simulink model "RTLAB_Sim_HVandLV_2015B"  (R2015b)
settings: Solver=ode45  StartTime=0.0  StopTime=20  RelTol=1e-3
values from neighbouring files (symbols this model uses):
  Ts = 20e-6    (= 2e-05)    [DataPostProcess.m]    (also in PlotData.m = 5e-05; data_analysis_01_MAT_load.m; data_analysis_01_Plot_result.m = 5e-05; data_analysis_02_Postprocess_Batch.m)
  Vrms_ph_hv = 37e3    (= 37000)    [DataPostProcess.m]    (also in data_analysis_01_MAT_load.m; data_analysis_05_Postprocess_Batch.m)
  Vrms_ph_lv = 690    [DataPostProcess.m]    (also in data_analysis_01_MAT_load.m; data_analysis_05_Postprocess_Batch.m)
libraries: powerlib_extras x5, powerlib_meascontrol x4, powerlib x1
settings Model: SimulationMode=accelerator  Creator=keliang  LastModifiedBy=anony
settings DataIOCC: SaveFormat=Array
settings OptimizationCC: EfficientMapNaN2IntZero=off
settings DebuggingCC: AllowSymbolicDim=on
settings HardwareCC: ProdWordSize=32  ProdHWDeviceType=Specified  TargetBitPerPointer=64  TargetLongLongMode=on  TargetIntDivRoundTo=Zero  TargetEndianess=LittleEndian  TargetWordSize=64  TargetHWDeviceType=MATLAB Host  ProdEqTarget=off
settings CodeAppCC: MaxIdLength=128
settings GRTTargetCC: CombineOutputUpdateFcns=off  GRTInterface=on
settings ConfigComp: CovModelRefEnable=Off
settings ConfigurationSet: Description=Simscape Multibody

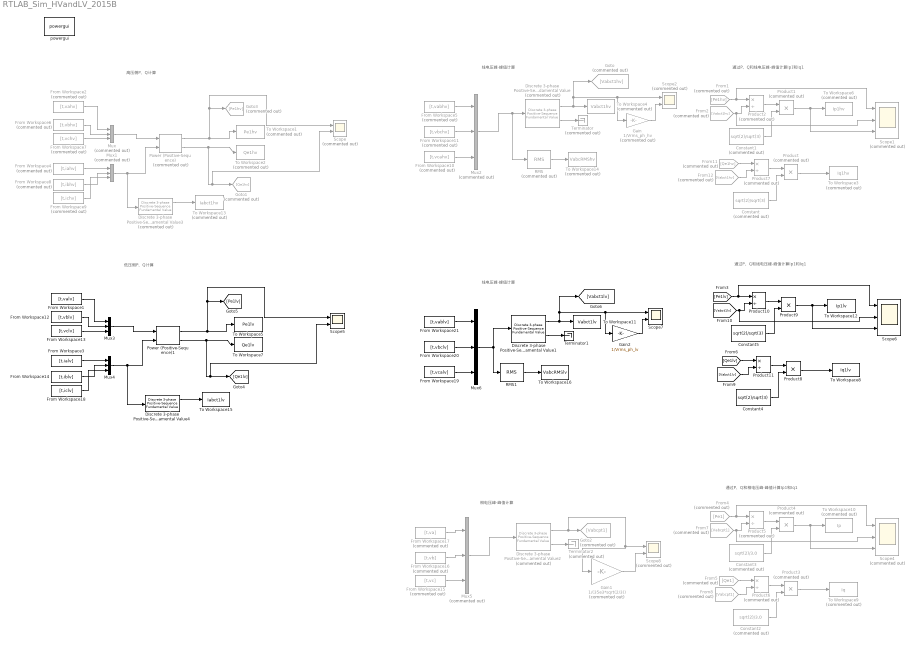
== system RTLAB_Sim_HVandLV_2015B ==
  note: 相电压峰-峰值计算
  note: 线电压峰-峰值计算
  note: 高压侧P、Q计算
  note: 通过P、Q和线电压峰-峰值计算Ip1和Iq1
  note: 通过P、Q和相电压峰-峰值计算Ip1和Iq1
  note: 低压侧P、Q计算
  note: 线电压峰-峰值计算
  note: 通过P、Q和线电压峰-峰值计算Ip1和Iq1
  Constant : Constant  Commented=on  Value=sqrt(2)/sqrt(3)
  Constant1 : Constant  Commented=on  Value=sqrt(2)/sqrt(3)
  Constant2 : Constant  Commented=on  Value=sqrt(2)/3.0
  Constant3 : Constant  Commented=on  Value=sqrt(2)/3.0
  Constant4 : Constant  Value=sqrt(2)/sqrt(3)
  Constant5 : Constant  Value=sqrt(2)/sqrt(3)
  Discrete 3-phase Positive-Sequence Fundamental Value : powerlib_extras/Discrete Measurements/Discrete 3-phase Positive-Sequence Fundamental Value  Commented=on  Freq=50  Par_Init=[0 0]  Ts=Ts
  Discrete 3-phase Positive-Sequence Fundamental Value1 : powerlib_extras/Discrete Measurements/Discrete 3-phase Positive-Sequence Fundamental Value  Freq=50  Par_Init=[0 0]  Ts=Ts
  Discrete 3-phase Positive-Sequence Fundamental Value2 : powerlib_extras/Discrete Measurements/Discrete 3-phase Positive-Sequence Fundamental Value  Commented=on  Freq=50  Par_Init=[0 0]  Ts=Ts
  Discrete 3-phase Positive-Sequence Fundamental Value3 : powerlib_extras/Discrete Measurements/Discrete 3-phase Positive-Sequence Fundamental Value  Commented=on  Freq=50  Par_Init=[0 0]  Ts=Ts
  Discrete 3-phase Positive-Sequence Fundamental Value4 : powerlib_extras/Discrete Measurements/Discrete 3-phase Positive-Sequence Fundamental Value  Freq=100  Par_Init=[0 0]  Ts=Ts
  From Workspace1 : FromWorkspace  VariableName=[t,valv]
  From Workspace10 : FromWorkspace  Commented=on  VariableName=[t,vcahv]
  From Workspace11 : FromWorkspace  Commented=on  VariableName=[t,vbchv]
  From Workspace12 : FromWorkspace  VariableName=[t,vblv]
  From Workspace13 : FromWorkspace  VariableName=[t,vclv]
  From Workspace14 : FromWorkspace  VariableName=[t,iblv]
  From Workspace15 : FromWorkspace  Commented=on  VariableName=[t,vc]
  From Workspace16 : FromWorkspace  Commented=on  VariableName=[t,vb]
  From Workspace17 : FromWorkspace  Commented=on  VariableName=[t,va]
  From Workspace18 : FromWorkspace  VariableName=[t,iclv]
  From Workspace19 : FromWorkspace  VariableName=[t,vcalv]
  From Workspace2 : FromWorkspace  Commented=on  VariableName=[t,vahv]
  From Workspace20 : FromWorkspace  VariableName=[t,vbclv]
  From Workspace21 : FromWorkspace  VariableName=[t,vablv]
  From Workspace3 : FromWorkspace  VariableName=[t,ialv]
  From Workspace4 : FromWorkspace  Commented=on  VariableName=[t,iahv]
  From Workspace5 : FromWorkspace  Commented=on  VariableName=[t,vabhv]
  From Workspace6 : FromWorkspace  Commented=on  VariableName=[t,vbhv]
  From Workspace7 : FromWorkspace  Commented=on  VariableName=[t,vchv]
  From Workspace8 : FromWorkspace  Commented=on  VariableName=[t,ibhv]
  From Workspace9 : FromWorkspace  Commented=on  VariableName=[t,ichv]
  From1 : From  Commented=on  GotoTag=Pe1hv
      settings: CloseFcn=tagdialog Close
  From11 : From  Commented=on  GotoTag=Qe1hv
      settings: CloseFcn=tagdialog Close
  From12 : From  Commented=on  GotoTag=Vabct1hv
      settings: CloseFcn=tagdialog Close
  From2 : From  Commented=on  GotoTag=Vabct1hv
      settings: CloseFcn=tagdialog Close
  From4 : From  Commented=on  GotoTag=Pe1
      settings: CloseFcn=tagdialog Close
  From5 : From  Commented=on  GotoTag=Qe1
      settings: CloseFcn=tagdialog Close
  From7 : From  Commented=on  GotoTag=Vabcpt1
      settings: CloseFcn=tagdialog Close
  From8 : From  Commented=on  GotoTag=Vabcpt1
      settings: CloseFcn=tagdialog Close
  Gain : Gain  Commented=on  Gain=1/Vrms_ph_hv
  Gain1 : Gain  Commented=on  Gain=1/(35e3*sqrt(2/3))
  Gain2 : Gain  Gain=1/Vrms_ph_lv
  Goto : Goto  Commented=on  GotoTag=Vabct1hv
  Goto1 : Goto  Commented=on  GotoTag=Qe1hv
  Goto2 : Goto  Commented=on  GotoTag=Vabcpt1
  Goto3 : Goto  Commented=on  GotoTag=Pe1hv
  Mux{,1..2,5} (4 alike) : Mux  Commented=on  Inputs=3
  Mux3 : Mux  Inputs=3
  Mux4 : Mux  Inputs=3
  Mux6 : Mux  Inputs=3
  Power (Positive-Sequence) : powerlib_meascontrol/Measurements/Power (Positive-Sequence)  Commented=on  Freq=50  Vinit=[0, 0]  Iinit=[0, 0]  Ts=Ts
  Power (Positive-Sequence)1 : powerlib_meascontrol/Measurements/Power (Positive-Sequence)  Freq=50  Vinit=[0, 0]  Iinit=[0, 0]  Ts=Ts
  Product{,1,3..4} (4 alike) : Product  Commented=on
  Product10 : Product  Inputs=*/  RndMeth=Zero
  Product11 : Product  Inputs=*/  RndMeth=Zero
  Product{2,5..7} (4 alike) : Product  Commented=on  Inputs=*/  RndMeth=Zero
  Product8 : Product
  Product9 : Product
  RMS : powerlib_meascontrol/Measurements/RMS  Commented=on  TrueRMS=on  Freq=100  RMSInit=0  Ts=Ts
  RMS1 : powerlib_meascontrol/Measurements/RMS  TrueRMS=on  Freq=100  RMSInit=0  Ts=Ts
  Scope : Scope  Commented=on  NumInputPorts=2
  Scope1 : Scope  Commented=on  NumInputPorts=3
  Scope2 : Scope  Commented=on  NumInputPorts=2
  Scope4 : Scope  Commented=on  NumInputPorts=3
  Scope5 : Scope  NumInputPorts=2
  Scope6 : Scope  NumInputPorts=3
  Scope7 : Scope  NumInputPorts=2
  Scope8 : Scope  Commented=on  NumInputPorts=2
  Terminator : Terminator  Commented=on
  Terminator1 : Terminator
  Terminator2 : Terminator  Commented=on
  To Workspace1 : ToWorkspace  Commented=on  VariableName=Pe1hv  SaveFormat=Structure With Time  SampleTime=-1
  To Workspace10 : ToWorkspace  Commented=on  VariableName=Ip  SaveFormat=Structure With Time  SampleTime=-1
  To Workspace11 : ToWorkspace  VariableName=Vabct1lv  SaveFormat=Structure With Time  SampleTime=-1
  To Workspace12 : ToWorkspace  VariableName=Ip1lv  SaveFormat=Structure With Time  SampleTime=-1
  To Workspace13 : ToWorkspace  Commented=on  VariableName=Iabct1hv  SaveFormat=Structure With Time  SampleTime=-1
  To Workspace14 : ToWorkspace  Commented=on  VariableName=VabcRMShv  SaveFormat=Structure With Time  SampleTime=-1
  To Workspace15 : ToWorkspace  VariableName=Iabct1lv  SaveFormat=Structure With Time  SampleTime=-1
  To Workspace16 : ToWorkspace  VariableName=VabcRMSlv  SaveFormat=Structure With Time  SampleTime=-1
  To Workspace2 : ToWorkspace  Commented=on  VariableName=Qe1hv  SaveFormat=Structure With Time  SampleTime=-1
  To Workspace3 : ToWorkspace  Commented=on  VariableName=Iq1hv  SaveFormat=Structure With Time  SampleTime=-1
  To Workspace4 : ToWorkspace  Commented=on  VariableName=Vabct1hv  SaveFormat=Structure With Time  SampleTime=-1
  To Workspace5 : ToWorkspace  VariableName=Pe1lv  SaveFormat=Structure With Time  SampleTime=-1
  To Workspace6 : ToWorkspace  Commented=on  VariableName=Ip1hv  SaveFormat=Structure With Time  SampleTime=-1
  To Workspace7 : ToWorkspace  VariableName=Qe1lv  SaveFormat=Structure With Time  SampleTime=-1
  To Workspace8 : ToWorkspace  VariableName=Iq1lv  SaveFormat=Structure With Time  SampleTime=-1
  To Workspace9 : ToWorkspace  Commented=on  VariableName=Iq  SaveFormat=Structure With Time  SampleTime=-1
  powergui : powerlib/powergui  Priority=1  SimulationMode=Discrete  SampleTime=Ts  frequency=60  Iterations=50  frequencyindice=60  Pbase=100e6  ErrMax=1e-4  UnitsV=kV  UnitsW=MW  buscounter=0  FunctionMessages=off  echomessages=off  EnableUseOfTLC=off  CurrentSourceSwitches=off  DisableSnubberDevices=off  DisableRonSwitches=off  DisableVfSwitches=off  DisplayEquations=off  AutomaticDiscreteSolvers=off  SolverType=Tustin  Interpol=off  ExternalGateDelay=off  methode=off  Ts=10  x0status=blocks  SPID=off  SwTol=0  HookPort=off  NonlinearTolerance=1e-4  nMaxIteration=100  ContinueOnMaxIteration=off  RestoreLinks=warning  ResistiveCurrentMeasurement=off  Frange=[0:2:500]  Ylog=off  Xlog=on  ShowGrid=off  save=off  variable=ZData  structure=v1  ZoomFFT=off  StartTime=3  cycles=50  DisplayStyle=1  fundamental=50  FreqAxis=off  MaxFrequency=2000  frequencyindicesteady=1  RmsSteady=1  display=off
  wires:
  Power (Positive-Sequence)/1 -> Scope/1, Goto3/1, To Workspace1/1
  Power (Positive-Sequence)/2 -> Scope/2, Goto1/1, To Workspace2/1
  From11/1 -> Product7/1
  From12/1 -> Product7/2
  Product7/1 -> Product/1
  Constant/1 -> Product/2
  Product/1 -> To Workspace3/1
  Discrete 3-phase Positive-Sequence Fundamental Value/2 -> Terminator/1
  Discrete 3-phase Positive-Sequence Fundamental Value/1 -> Gain/1, Scope2/1, Goto/1, To Workspace4/1
  Mux/1 -> Power (Positive-Sequence)/1
  Mux1/1 -> Power (Positive-Sequence)/2, Discrete 3-phase Positive-Sequence Fundamental Value3/1
  From Workspace2/1 -> Mux/1
  From Workspace6/1 -> Mux/2
  From Workspace7/1 -> Mux/3
  From Workspace4/1 -> Mux1/1
  From Workspace8/1 -> Mux1/2
  From Workspace9/1 -> Mux1/3
  From Workspace5/1 -> Mux2/1
  From Workspace11/1 -> Mux2/2
  From Workspace10/1 -> Mux2/3
  Mux2/1 -> RMS/1, Discrete 3-phase Positive-Sequence Fundamental Value/1
  Discrete 3-phase Positive-Sequence Fundamental Value2/2 -> Terminator2/1
  Discrete 3-phase Positive-Sequence Fundamental Value2/1 -> Gain1/1, Scope8/1, Goto2/1
  From Workspace17/1 -> Mux5/1
  From Workspace16/1 -> Mux5/2
  From Workspace15/1 -> Mux5/3
  Mux5/1 -> Discrete 3-phase Positive-Sequence Fundamental Value2/1
  From1/1 -> Scope1/1, Product2/1
  From2/1 -> Scope1/2, Product2/2
  Product2/1 -> Product1/1
  Constant1/1 -> Product1/2
  Product1/1 -> Scope1/3, To Workspace6/1
  Constant3/1 -> Product4/2
  Product5/1 -> Product4/1
  Product4/1 -> Scope4/3, To Workspace10/1
  Product3/1 -> To Workspace9/1
  From8/1 -> Product6/2
  From7/1 -> Scope4/2, Product5/2
  From5/1 -> Product6/1
  From4/1 -> Scope4/1, Product5/1
  Constant2/1 -> Product3/2
  Product6/1 -> Product3/1
  Power (Positive-Sequence)1/1 -> Scope5/1, [Pe1lv], To Workspace5/1
  From Workspace14/1 -> Mux4/2
  From Workspace18/1 -> Mux4/3
  Power (Positive-Sequence)1/2 -> Scope5/2, [Qe1lv], To Workspace7/1
  From Workspace1/1 -> Mux3/1
  From Workspace12/1 -> Mux3/2
  Mux3/1 -> Power (Positive-Sequence)1/1
  From Workspace13/1 -> Mux3/3
  From Workspace3/1 -> Mux4/1
  Mux4/1 -> Discrete 3-phase Positive-Sequence Fundamental Value4/1, Power (Positive-Sequence)1/2
  Product9/1 -> To Workspace12/1, Scope6/3
  Constant5/1 -> Product9/2
  Product10/1 -> Product9/1
  [Vabct1lv] -> Product10/2, Scope6/2
  [Pe1lv] -> Product10/1, Scope6/1
  Mux6/1 -> Discrete 3-phase Positive-Sequence Fundamental Value1/1, RMS1/1
  From Workspace19/1 -> Mux6/3
  From Workspace20/1 -> Mux6/2
  From Workspace21/1 -> Mux6/1
  Discrete 3-phase Positive-Sequence Fundamental Value1/1 -> To Workspace11/1, [Vabct1lv], Gain2/1, Scope7/1
  Discrete 3-phase Positive-Sequence Fundamental Value1/2 -> Terminator1/1
  Product8/1 -> To Workspace8/1
  Constant4/1 -> Product8/2
  Product11/1 -> Product8/1
  [Vabct1lv] -> Product11/2
  [Qe1lv] -> Product11/1
  Gain/1 -> Scope2/2
  Gain1/1 -> Scope8/2
  Discrete 3-phase Positive-Sequence Fundamental Value3/1 -> To Workspace13/1
  RMS/1 -> To Workspace14/1
  Discrete 3-phase Positive-Sequence Fundamental Value4/1 -> To Workspace15/1
  Gain2/1 -> Scope7/2
  RMS1/1 -> To Workspace16/1
